simulink model "testmodel_1109"  (R2015b)
settings: Solver=FixedStepDiscrete  StartTime=0.0  StopTime=50  FixedStep=Ts  RelTol=1e-3
PreLoadFcn:
  | Ts_IO601 = 0.001;
InitFcn:
  | Ts_IO601 = 0.001;
  | Ts=0.004;
undefined symbols (not defined in the file or in its folder): DiscIntNeverNeededParam
libraries: canmsglib x13, speedgoatlib_IO601 x9, slrtlib x5, simulink x3
settings Model: Creator=lab2  LastModifiedBy=mohit
settings SolverCC: EnableConcurrentExecution=on
settings DataIOCC: SaveFormat=Array
settings OptimizationCC: BlockReduction=off  OptimizeBlockIOStorage=off  BufferReuse=off  GlobalBufferReuse=off  ExpressionFolding=off  LocalBlockOutputs=off
settings DebuggingCC: UnconnectedInputMsg=none  UnconnectedOutputMsg=none  UnconnectedLineMsg=none
settings HardwareCC: ProdBitPerPointer=32  ProdLargestAtomicFloat=None  ProdWordSize=32  ProdLongLongMode=on  ProdHWDeviceType=Generic->32-bit x86 compatible
settings RTWCC: SystemTargetFile=slrt.tlc  TemplateMakefile=slrt_default_tmf  Description=Simulink Real-Time  RTWCompilerOptimization=on
settings TargetCC: CodeReplacementLibrary=XPC_BLAS  ParMdlRefBuildCompliant=on  ConcurrentExecutionCompliant=on  GeneratePreprocessorConditionals=Use local settings  MatFileLogging=on  MATLABClassNameForMDSCustomization=xpcAperiodicCustomization
settings ConfigComp: CovModelRefEnable=Off

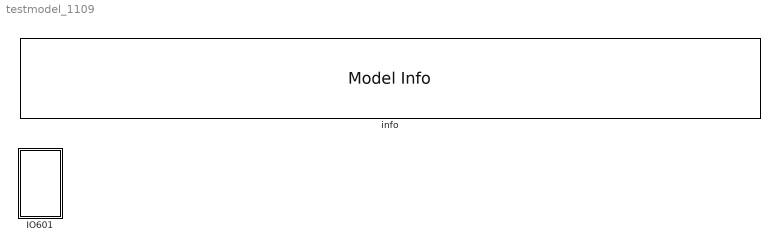
== system testmodel_1109 ==
  IO601 : Subsystem
  info : simulink/Model-Wide Utilities/Model Info  Frame=on  DisplayStringWithTags=|  HorizontalTextAlignment=Left  LeftAlignmentValue=0.02  SourceBlockDiagram=testmodel_1109  TagMaxNumber=20
      | SPEEDGOAT Simulink Real-Time  test model for Real-time target machine (SN2820)
      | prepared by Speedgoat with MATLAB R2015a
      | 
      | Build date: %<Created>

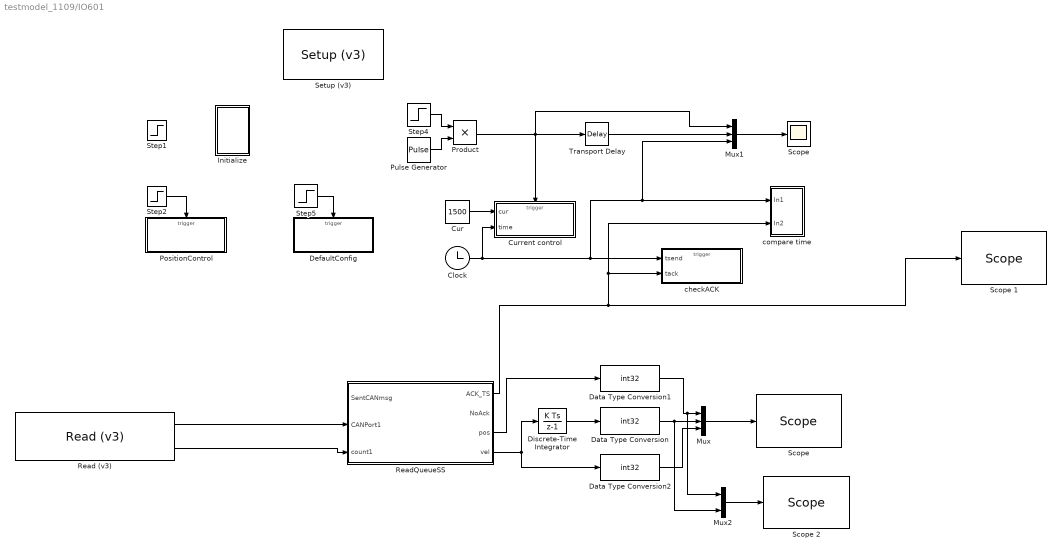
== system testmodel_1109/IO601 ==
  Clock : Clock
  Cur : Constant  Value=1500  OutMin=-1500  OutMax=1500  OutDataTypeStr=int32
  Current control : Subsystem  TreatAsAtomicUnit=on
  Data Type Conversion : DataTypeConversion  OutDataTypeStr=int32
  Data Type Conversion1 : DataTypeConversion  OutDataTypeStr=int32
  Data Type Conversion2 : DataTypeConversion  OutDataTypeStr=int32
  DefaultConfig : Subsystem  TreatAsAtomicUnit=on
  Discrete-Time Integrator : DiscreteIntegrator  InitialConditionSetting=State (most efficient)  SampleTime=-1  ICPrevOutput=DiscIntNeverNeededParam  ICPrevScaledInput=DiscIntNeverNeededParam
  Initialize : Subsystem
  Mux : Mux  Inputs=3
  Mux1 : Mux  Inputs=3
  Mux2 : Mux  Inputs=2
  "PositionControl " : Subsystem  TreatAsAtomicUnit=on
  Product : Product
  Pulse Generator : DiscretePulseGenerator  PulseType=Time based  Period=Ts*10  PulseWidth=10  PhaseDelay=10  SampleTime=Ts_IO601
  Read (v3) : speedgoatlib_IO601/Read (v3)  id=1  outputFormat=Vector of CAN_MESSAGE  port1=on  port2=off  depth1=37  depth2=4  sampletime=Ts  pciSlot=-1
  ReadQueueSS : Subsystem
  Scope : Scope
  "Scope " : slrtlib/Displays and Logging/Scope   scopeno=3  scopetype=Target  autostart=on  viewmode=Graphical sliding  formatstr='%15.6f'  grid=on  ylimits=[-90000,90000]  nosamples=50/Ts  noprepostsamples=0  interleave=1  triggermode=FreeRun  triggersignal=1  trigsignalfromport=off  triggerlevel=0.0  triggerslope=Either  triggerscope=1  triggersample=0  filename=data.dat  mode=Lazy  writesize=512  autorestart=off  dynamicfilemode=off  maxwritefilesize=512*1024^2
  Scope 1 : slrtlib/Displays and Logging/Scope   scopeno=12  scopetype=Target  autostart=on  viewmode=Graphical sliding  formatstr='%15.6f'  grid=on  ylimits=[0,125000]  nosamples=50/Ts  noprepostsamples=0  interleave=1  triggermode=FreeRun  triggersignal=1  trigsignalfromport=on  triggerlevel=0.0  triggerslope=Either  triggerscope=1  triggersample=0  filename=data.dat  mode=Lazy  writesize=512  autorestart=off  dynamicfilemode=off  maxwritefilesize=512*1024^2
  Scope 2 : slrtlib/Displays and Logging/Scope   scopeno=1  scopetype=File  autostart=on  viewmode=Graphical sliding  formatstr='%15.6f'  grid=on  ylimits=[-90000,90000]  nosamples=50/Ts  noprepostsamples=0  interleave=1  triggermode=FreeRun  triggersignal=1  trigsignalfromport=off  triggerlevel=0.0  triggerslope=Either  triggerscope=1  triggersample=0  filename=pos_vel.dat  mode=Lazy  writesize=512  autorestart=off  dynamicfilemode=off  maxwritefilesize=512*1024^2
  Setup (v3) : speedgoatlib_IO601/Setup (v3)  id=1  can1enable=on  can1bus=Highspeed  can1Baudrate=1 MBaud  can1UserBR=[1,1,5,2]  stdAcc1=[0,0,0,0]  extAcc1=[0,0,0,0]  can2enable=on  can2bus=Highspeed  can2Baudrate=1 MBaud  can2UserBR=[1,1,5,2]  stdAcc2=[0,0,0,0]  extAcc2=[0,0,0,0]  pciSlot=-1
  Step1 : Step  Time=10  SampleTime=Ts
  Step2 : Step  Time=25  SampleTime=Ts
  Step4 : Step  Time=14  Before=1  After=0  SampleTime=0
  Step5 : Step  Time=15  SampleTime=Ts
  Transport Delay : TransportDelay  DelayTime=Ts*10
  checkACK : Subsystem
  compare time : Subsystem
  wires:
  Step4/1 -> Product/1
  Pulse Generator/1 -> Product/2
  ReadQueueSS/1(ACK_TS) -> compare time/2(In2), checkACK/2(tack), Scope 1/1
  Cur/1 -> Current control/1(cur)
  Read (v3)/1 -> ReadQueueSS/2(CANPort1)
  Read (v3)/2 -> ReadQueueSS/3(count1)
  Step2/1 -> "PositionControl "/Trigger
  Product/1 -> Mux1/1, Transport Delay/1, Current control/Trigger
  Clock/1 -> Mux1/3, compare time/1(In1), checkACK/1(tsend), Current control/2(time)
  ReadQueueSS/4(vel) -> Discrete-Time Integrator/1, Data Type Conversion2/1
  Mux/1 -> "Scope "/1
  Discrete-Time Integrator/1 -> Data Type Conversion/1
  Data Type Conversion/1 -> Mux2/2, Mux/2
  Data Type Conversion1/1 -> Mux2/1, Mux/1
  Data Type Conversion2/1 -> Mux/3
  Transport Delay/1 -> Mux1/2
  Mux1/1 -> Scope/1
  Mux2/1 -> Scope 2/1
  ReadQueueSS/3(pos) -> Data Type Conversion1/1
  Step5/1 -> DefaultConfig/Trigger

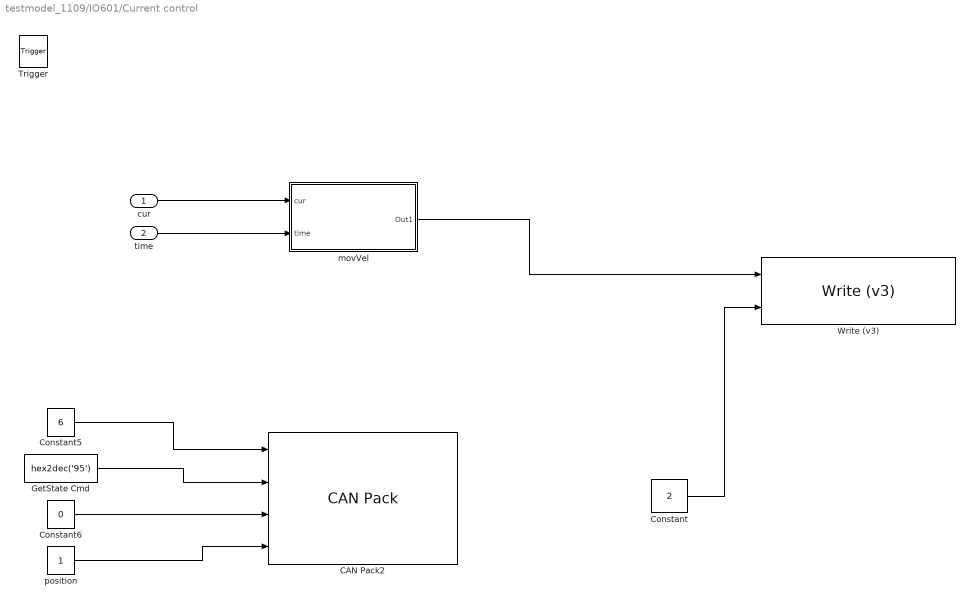
== system testmodel_1109/IO601/Current control ==
  cur : Inport
  time : Inport  Port=2
  Trigger : TriggerPort
  CAN Pack2 : canmsglib/CAN Pack  MsgList=(none)  MsgName=GetState  MsgIDType=Standard (11-bit identifier)  MsgIdentifier=hex2dec('503')  MsgLength=7  SignalInfo=Signal1$0$8$1$2$1$0$1$0$-Inf$Inf$#Signal2$8$8$1$2$1$0$1$0$-Inf$Inf$#time$16$32$1$2$1$0$1$0$-Inf$Inf$#mode$48$8$1$2$1$0$1$0$-Inf$Inf$#  NSignals=4  StartBits=str2num('[int32(0);int32(8);int32(16);int32(48)]')  SignalSizes=str2num('[int32(8);int32(8);int32(32);int32(8)]')  ByteOrders=str2num('[int32(1);int32(1);int32(1);int32(1)]')  DataTypes=str2num('[int32(2);int32(2);int32(2);int32(2)]')  MultiplexTypes=str2num('[int32(1);int32(1);int32(1);int32(1)]')  MultiplexValues=str2num('[double(0);double(0);double(0);double(0)]')  Factors=str2num('[double(1);double(1);double(1);double(1)]')  Offsets=str2num('[double(0);double(0);double(0);double(0)]')  Minimums=str2num('[double(-Inf);double(-Inf);double(-Inf);double(-Inf)]')  Maximums=str2num('[double(Inf);double(Inf);double(Inf);double(Inf)]')  Remote=off
      settings: DataFormat=manually specified signals
  Constant : Constant  Value=2
  Constant5 : Constant  Value=6
  Constant6 : Constant  Value=0
  GetState Cmd : Constant  Value=hex2dec('95')
  Write (v3) : speedgoatlib_IO601/Write (v3)  Priority=1  id=1  sampletime=-1  pciSlot=-1  inputType=CAN_MESSAGE plus count  port=1  maxMsg=2  status=on  init=[]  term=[]
  movVel : Subsystem
  position : Constant  OutDataTypeStr=uint8
  wires:
  Constant/1 -> Write (v3)/2
  Constant6/1 -> CAN Pack2/3
  Constant5/1 -> CAN Pack2/1
  GetState Cmd/1 -> CAN Pack2/2
  position/1 -> CAN Pack2/4
  cur/1 -> movVel/1(cur)
  time/1 -> movVel/2(time)
  movVel/1(Out1) -> Write (v3)/1

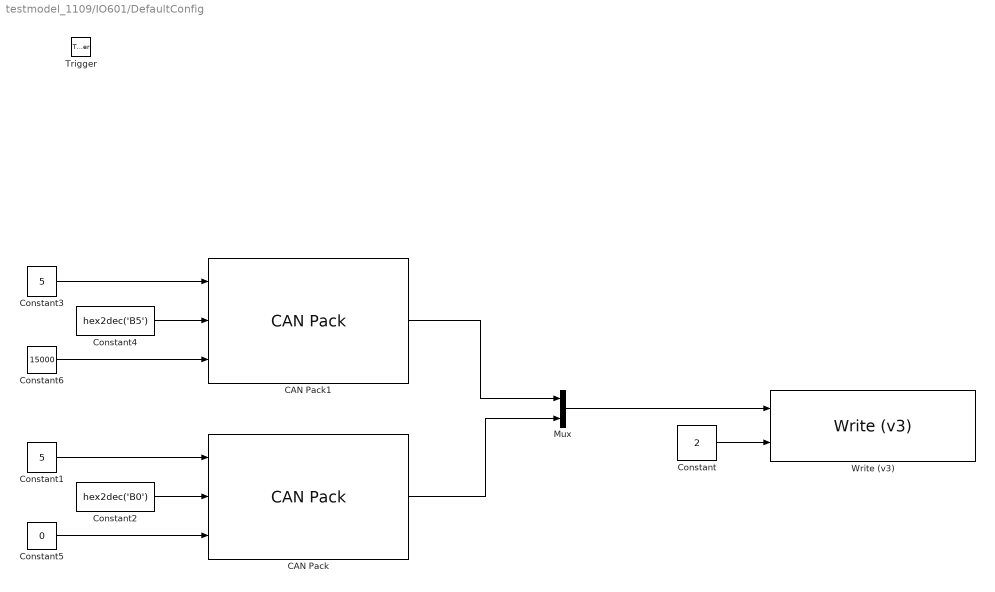
== system testmodel_1109/IO601/DefaultConfig ==
  Trigger : TriggerPort
  CAN Pack : canmsglib/CAN Pack  MsgList=(none)  MsgName=Position Msg  MsgIDType=Standard (11-bit identifier)  MsgIdentifier=hex2dec('503')  MsgLength=6  SignalInfo=Signal1$0$8$1$2$1$0$1$0$-Inf$Inf$#Signal2$8$8$1$2$1$0$1$0$-Inf$Inf$#Signal3$16$32$1$1$1$0$1$0$-Inf$Inf$#  NSignals=3  StartBits=str2num('[int32(0);int32(8);int32(16)]')  SignalSizes=str2num('[int32(8);int32(8);int32(32)]')  ByteOrders=str2num('[int32(1);int32(1);int32(1)]')  DataTypes=str2num('[int32(2);int32(2);int32(1)]')  MultiplexTypes=str2num('[int32(1);int32(1);int32(1)]')  MultiplexValues=str2num('[double(0);double(0);double(0)]')  Factors=str2num('[double(1);double(1);double(1)]')  Offsets=str2num('[double(0);double(0);double(0)]')  Minimums=str2num('[double(-Inf);double(-Inf);double(-Inf)]')  Maximums=str2num('[double(Inf);double(Inf);double(Inf)]')  Remote=off
      settings: DataFormat=manually specified signals
  CAN Pack1 : canmsglib/CAN Pack  MsgList=(none)  MsgName=Position Msg  MsgIDType=Standard (11-bit identifier)  MsgIdentifier=hex2dec('503')  MsgLength=6  SignalInfo=Signal1$0$8$1$2$1$0$1$0$-Inf$Inf$#Signal2$8$8$1$2$1$0$1$0$-Inf$Inf$#Signal3$16$32$1$1$1$0$1$0$-Inf$Inf$#  NSignals=3  StartBits=str2num('[int32(0);int32(8);int32(16)]')  SignalSizes=str2num('[int32(8);int32(8);int32(32)]')  ByteOrders=str2num('[int32(1);int32(1);int32(1)]')  DataTypes=str2num('[int32(2);int32(2);int32(1)]')  MultiplexTypes=str2num('[int32(1);int32(1);int32(1)]')  MultiplexValues=str2num('[double(0);double(0);double(0)]')  Factors=str2num('[double(1);double(1);double(1)]')  Offsets=str2num('[double(0);double(0);double(0)]')  Minimums=str2num('[double(-Inf);double(-Inf);double(-Inf)]')  Maximums=str2num('[double(Inf);double(Inf);double(Inf)]')  Remote=off
      settings: DataFormat=manually specified signals
  Constant : Constant  Value=2
  Constant1 : Constant  Value=5
  Constant2 : Constant  Value=hex2dec('B0')
  Constant3 : Constant  Value=5
  Constant4 : Constant  Value=hex2dec('B5')
  Constant5 : Constant  Value=0
  Constant6 : Constant  Value=15000
  Mux : Mux  Inputs=2
  Write (v3) : speedgoatlib_IO601/Write (v3)  Priority=1  id=1  sampletime=-1  pciSlot=-1  inputType=CAN_MESSAGE plus count  port=1  maxMsg=2  status=off  init=[]  term=[]
  wires:
  CAN Pack/1 -> Mux/2
  Constant/1 -> Write (v3)/2
  Constant1/1 -> CAN Pack/1
  Constant2/1 -> CAN Pack/2
  Constant5/1 -> CAN Pack/3
  CAN Pack1/1 -> Mux/1
  Constant3/1 -> CAN Pack1/1
  Constant4/1 -> CAN Pack1/2
  Constant6/1 -> CAN Pack1/3
  Mux/1 -> Write (v3)/1

== system testmodel_1109/IO601/Initialize ==
  GetState(ms) : Subsystem  TreatAsAtomicUnit=on
  InitialPosition : Subsystem  TreatAsAtomicUnit=on
  QuitError : Subsystem  TreatAsAtomicUnit=on
  Step : Step  SampleTime=Ts
  Step1 : Step  Time=2  SampleTime=Ts
  Step3 : Step  Time=2  SampleTime=Ts
  wires:
  Step/1 -> QuitError/Trigger
  Step3/1 -> InitialPosition/Trigger
  Step1/1 -> GetState(ms)/Trigger

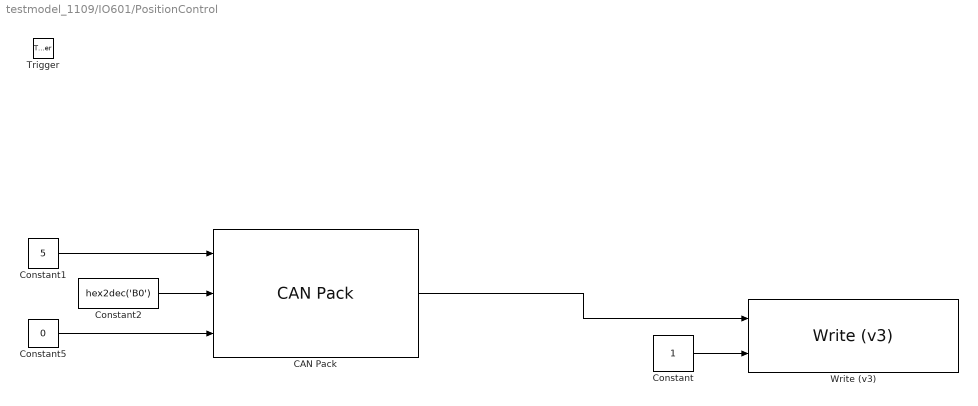
== system testmodel_1109/IO601/PositionControl  ==
  Trigger : TriggerPort
  CAN Pack : canmsglib/CAN Pack  MsgList=(none)  MsgName=Position Msg  MsgIDType=Standard (11-bit identifier)  MsgIdentifier=hex2dec('503')  MsgLength=6  SignalInfo=Signal1$0$8$1$2$1$0$1$0$-Inf$Inf$#Signal2$8$8$1$2$1$0$1$0$-Inf$Inf$#Signal3$16$32$1$1$1$0$1$0$-Inf$Inf$#  NSignals=3  StartBits=str2num('[int32(0);int32(8);int32(16)]')  SignalSizes=str2num('[int32(8);int32(8);int32(32)]')  ByteOrders=str2num('[int32(1);int32(1);int32(1)]')  DataTypes=str2num('[int32(2);int32(2);int32(1)]')  MultiplexTypes=str2num('[int32(1);int32(1);int32(1)]')  MultiplexValues=str2num('[double(0);double(0);double(0)]')  Factors=str2num('[double(1);double(1);double(1)]')  Offsets=str2num('[double(0);double(0);double(0)]')  Minimums=str2num('[double(-Inf);double(-Inf);double(-Inf)]')  Maximums=str2num('[double(Inf);double(Inf);double(Inf)]')  Remote=off
      settings: DataFormat=manually specified signals
  Constant : Constant
  Constant1 : Constant  Value=5
  Constant2 : Constant  Value=hex2dec('B0')
  Constant5 : Constant  Value=0
  Write (v3) : speedgoatlib_IO601/Write (v3)  Priority=1  id=1  sampletime=-1  pciSlot=-1  inputType=CAN_MESSAGE plus count  port=1  maxMsg=1  status=off  init=[]  term=[]
  wires:
  CAN Pack/1 -> Write (v3)/1
  Constant/1 -> Write (v3)/2
  Constant1/1 -> CAN Pack/1
  Constant2/1 -> CAN Pack/2
  Constant5/1 -> CAN Pack/3

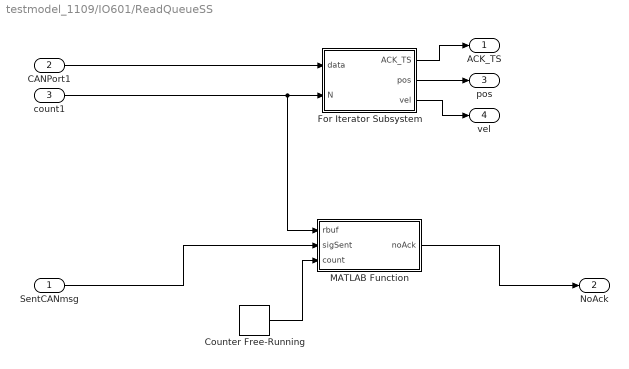
== system testmodel_1109/IO601/ReadQueueSS ==
  SentCANmsg : Inport
  CANPort1 : Inport  Port=2
  count1 : Inport  Port=3
  Counter Free-Running : simulink/Sources/Counter Free-Running  NumBits=2  tsamp=-1
  For Iterator Subsystem : Subsystem  TreatAsAtomicUnit=on
  MATLAB Function : MATLAB Function  TreatAsAtomicUnit=on
  ACK_TS : Outport
  " NoAck" : Outport  Port=2
  pos : Outport  Port=3
  vel : Outport  Port=4
  wires:
  CANPort1/1 -> For Iterator Subsystem/1(data)
  count1/1 -> MATLAB Function/1(rbuf), For Iterator Subsystem/2(N)
  For Iterator Subsystem/1(ACK_TS) -> ACK_TS/1
  Counter Free-Running/1 -> MATLAB Function/3(count)
  SentCANmsg/1 -> MATLAB Function/2(sigSent)
  MATLAB Function/1(noAck) -> " NoAck"/1
  For Iterator Subsystem/2(pos) -> pos/1
  For Iterator Subsystem/3(vel) -> vel/1

== system testmodel_1109/IO601/checkACK ==
  tsend : Inport
  tack : Inport  Port=2
  Trigger : TriggerPort
  MATLAB Function : MATLAB Function  TreatAsAtomicUnit=on
  STOP : Subsystem  TreatAsAtomicUnit=on
  wires:
  MATLAB Function/1(stop) -> STOP/1(stop)
  tack/1 -> MATLAB Function/2(tack)
  tsend/1 -> MATLAB Function/1(tsend)

== system testmodel_1109/IO601/compare time ==
  In1 : Inport
  In2 : Inport  Port=2
  Mux2 : Mux  Inputs=2
  Scope 2 : slrtlib/Displays and Logging/Scope   scopeno=50  scopetype=Target  autostart=on  viewmode=Graphical sliding  formatstr='%15.6f'  grid=on  ylimits=[0,125000]  nosamples=50/Ts  noprepostsamples=0  interleave=1  triggermode=FreeRun  triggersignal=1  trigsignalfromport=on  triggerlevel=0.0  triggerslope=Either  triggerscope=1  triggersample=0  filename=data.dat  mode=Lazy  writesize=512  autorestart=off  dynamicfilemode=off  maxwritefilesize=512*1024^2
  wires:
  Mux2/1 -> Scope 2/1
  In1/1 -> Mux2/1
  In2/1 -> Mux2/2

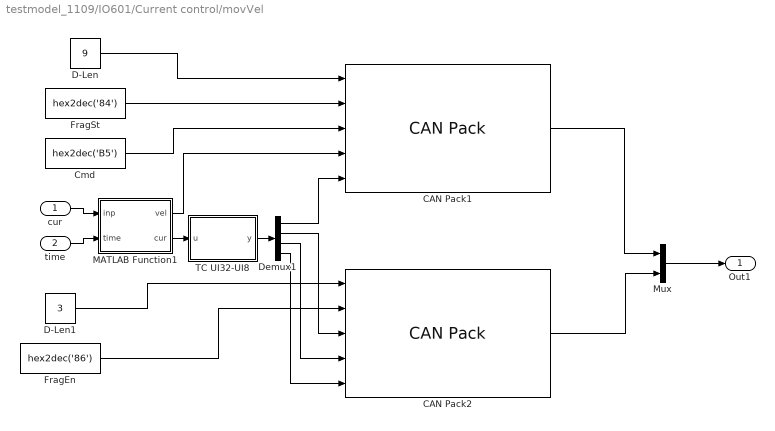
== system testmodel_1109/IO601/Current control/movVel ==
  cur : Inport
  time : Inport  Port=2
  CAN Pack1 : canmsglib/CAN Pack  MsgList=(none)  MsgName=Position Msg  MsgIDType=Standard (11-bit identifier)  MsgIdentifier=hex2dec('503')  MsgLength=8  SignalInfo=Signal1$0$8$1$2$1$0$1$0$-Inf$Inf$#Signal2$8$8$1$2$1$0$1$0$-Inf$Inf$#Signal3$16$8$1$2$1$0$1$0$-Inf$Inf$#Signal4$24$32$1$1$1$0$1$0$-Inf$Inf$#Signal5$56$8$1$2$1$0$1$0$-Inf$Inf$#  NSignals=5  StartBits=str2num('[int32(0);int32(8);int32(16);int32(24);int32(56)]')  SignalSizes=str2num('[int32(8);int32(8);int32(8);int32(32);int32(8)]')  ByteOrders=str2num('[int32(1);int32(1);int32(1);int32(1);int32(1)]')  DataTypes=str2num('[int32(2);int32(2);int32(2);int32(1);int32(2)]')  MultiplexTypes=str2num('[int32(1);int32(1);int32(1);int32(1);int32(1)]')  MultiplexValues=str2num('[double(0);double(0);double(0);double(0);double(0)]')  Factors=str2num('[double(1);double(1);double(1);double(1);double(1)]')  Offsets=str2num('[double(0);double(0);double(0);double(0);double(0)]')  Minimums=str2num('[double(-Inf);double(-Inf);double(-Inf);double(-Inf);double(-Inf)]')  Maximums=str2num('[double(Inf);double(Inf);double(Inf);double(Inf);double(Inf)]')  Remote=off
      settings: DataFormat=manually specified signals
  CAN Pack2 : canmsglib/CAN Pack  MsgList=(none)  MsgName=Position Msg  MsgIDType=Standard (11-bit identifier)  MsgIdentifier=hex2dec('503')  MsgLength=5  SignalInfo=Signal1$0$8$1$2$1$0$1$0$-Inf$Inf$#Signal2$8$8$1$2$1$0$1$0$-Inf$Inf$#Signal3$16$8$1$2$1$0$1$0$-Inf$Inf$#Signal4$24$8$1$2$1$0$1$0$-Inf$Inf$#Signal5$32$8$1$2$1$0$1$0$-Inf$Inf$#  NSignals=5  StartBits=str2num('[int32(0);int32(8);int32(16);int32(24);int32(32)]')  SignalSizes=str2num('[int32(8);int32(8);int32(8);int32(8);int32(8)]')  ByteOrders=str2num('[int32(1);int32(1);int32(1);int32(1);int32(1)]')  DataTypes=str2num('[int32(2);int32(2);int32(2);int32(2);int32(2)]')  MultiplexTypes=str2num('[int32(1);int32(1);int32(1);int32(1);int32(1)]')  MultiplexValues=str2num('[double(0);double(0);double(0);double(0);double(0)]')  Factors=str2num('[double(1);double(1);double(1);double(1);double(1)]')  Offsets=str2num('[double(0);double(0);double(0);double(0);double(0)]')  Minimums=str2num('[double(-Inf);double(-Inf);double(-Inf);double(-Inf);double(-Inf)]')  Maximums=str2num('[double(Inf);double(Inf);double(Inf);double(Inf);double(Inf)]')  Remote=off
      settings: DataFormat=manually specified signals
  Cmd : Constant  Value=hex2dec('B5')
  D-Len : Constant  Value=9
  D-Len1 : Constant  Value=3
  Demux1 : Demux
  FragEn : Constant  Value=hex2dec('86')
  FragSt : Constant  Value=hex2dec('84')
  MATLAB Function1 : MATLAB Function  TreatAsAtomicUnit=on
  Mux : Mux  Inputs=2
  TC UI32-UI8 : MATLAB Function  TreatAsAtomicUnit=on
  Out1 : Outport
  wires:
  D-Len/1 -> CAN Pack1/1
  Cmd/1 -> CAN Pack1/3
  CAN Pack1/1 -> Mux/1
  Mux/1 -> Out1/1
  FragSt/1 -> CAN Pack1/2
  FragEn/1 -> CAN Pack2/2
  D-Len1/1 -> CAN Pack2/1
  CAN Pack2/1 -> Mux/2
  MATLAB Function1/2(cur) -> TC UI32-UI8/1(u)
  Demux1/1 -> CAN Pack1/5
  Demux1/2 -> CAN Pack2/3
  Demux1/3 -> CAN Pack2/4
  Demux1/4 -> CAN Pack2/5
  cur/1 -> MATLAB Function1/1(inp)
  time/1 -> MATLAB Function1/2(time)
  MATLAB Function1/1(vel) -> CAN Pack1/4
  TC UI32-UI8/1(y) -> Demux1/1

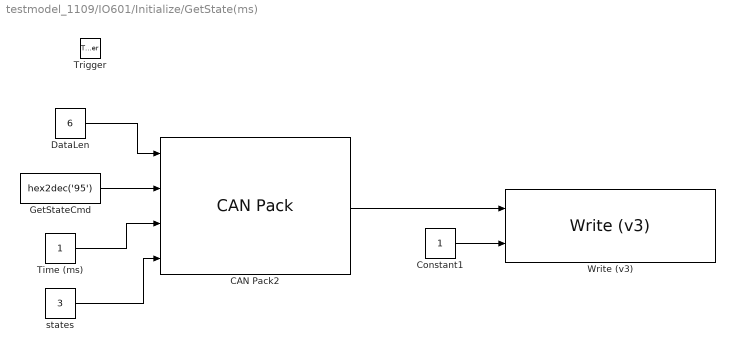
== system testmodel_1109/IO601/Initialize/GetState(ms) ==
  Trigger : TriggerPort
  CAN Pack2 : canmsglib/CAN Pack  MsgList=(none)  MsgName=GetState  MsgIDType=Standard (11-bit identifier)  MsgIdentifier=hex2dec('503')  MsgLength=7  SignalInfo=Signal1$0$8$1$2$1$0$1$0$-Inf$Inf$#Signal2$8$8$1$2$1$0$1$0$-Inf$Inf$#time$16$32$1$2$1$0$1$0$-Inf$Inf$#mode$48$8$1$2$1$0$1$0$-Inf$Inf$#  NSignals=4  StartBits=str2num('[int32(0);int32(8);int32(16);int32(48)]')  SignalSizes=str2num('[int32(8);int32(8);int32(32);int32(8)]')  ByteOrders=str2num('[int32(1);int32(1);int32(1);int32(1)]')  DataTypes=str2num('[int32(2);int32(2);int32(2);int32(2)]')  MultiplexTypes=str2num('[int32(1);int32(1);int32(1);int32(1)]')  MultiplexValues=str2num('[double(0);double(0);double(0);double(0)]')  Factors=str2num('[double(1);double(1);double(1);double(1)]')  Offsets=str2num('[double(0);double(0);double(0);double(0)]')  Minimums=str2num('[double(-Inf);double(-Inf);double(-Inf);double(-Inf)]')  Maximums=str2num('[double(Inf);double(Inf);double(Inf);double(Inf)]')  Remote=off
      settings: DataFormat=manually specified signals
  Constant1 : Constant
  DataLen : Constant  Value=6
  GetStateCmd : Constant  Value=hex2dec('95')
  Time (ms) : Constant
  Write (v3) : speedgoatlib_IO601/Write (v3)  Priority=1  id=1  sampletime=-1  pciSlot=-1  inputType=CAN_MESSAGE plus count  port=1  maxMsg=1  status=off  init=[]  term=[]
  states : Constant  Value=3  OutDataTypeStr=uint8
  wires:
  Constant1/1 -> Write (v3)/2
  Time (ms)/1 -> CAN Pack2/3
  DataLen/1 -> CAN Pack2/1
  GetStateCmd/1 -> CAN Pack2/2
  CAN Pack2/1 -> Write (v3)/1
  states/1 -> CAN Pack2/4

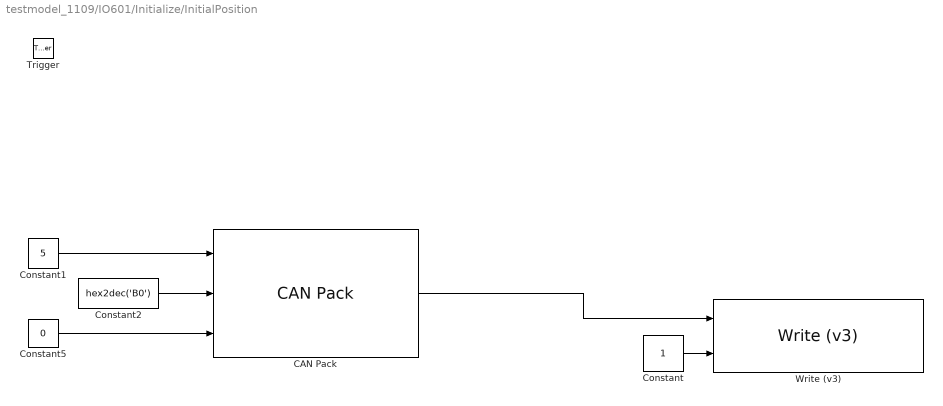
== system testmodel_1109/IO601/Initialize/InitialPosition ==
  Trigger : TriggerPort
  CAN Pack : canmsglib/CAN Pack  MsgList=(none)  MsgName=Position Msg  MsgIDType=Standard (11-bit identifier)  MsgIdentifier=1283  MsgLength=6  SignalInfo=Signal1$0$8$1$2$1$0$1$0$-Inf$Inf$#Signal2$8$8$1$2$1$0$1$0$-Inf$Inf$#Signal3$16$32$1$1$1$0$1$0$-Inf$Inf$#  NSignals=3  StartBits=str2num('[int32(0);int32(8);int32(16)]')  SignalSizes=str2num('[int32(8);int32(8);int32(32)]')  ByteOrders=str2num('[int32(1);int32(1);int32(1)]')  DataTypes=str2num('[int32(2);int32(2);int32(1)]')  MultiplexTypes=str2num('[int32(1);int32(1);int32(1)]')  MultiplexValues=str2num('[double(0);double(0);double(0)]')  Factors=str2num('[double(1);double(1);double(1)]')  Offsets=str2num('[double(0);double(0);double(0)]')  Minimums=str2num('[double(-Inf);double(-Inf);double(-Inf)]')  Maximums=str2num('[double(Inf);double(Inf);double(Inf)]')  Remote=off
      settings: DataFormat=manually specified signals
  Constant : Constant
  Constant1 : Constant  Value=5
  Constant2 : Constant  Value=hex2dec('B0')
  Constant5 : Constant  Value=0
  Write (v3) : speedgoatlib_IO601/Write (v3)  Priority=1  id=1  sampletime=-1  pciSlot=-1  inputType=CAN_MESSAGE plus count  port=1  maxMsg=1  status=off  init=[]  term=[]
  wires:
  CAN Pack/1 -> Write (v3)/1
  Constant/1 -> Write (v3)/2
  Constant1/1 -> CAN Pack/1
  Constant2/1 -> CAN Pack/2
  Constant5/1 -> CAN Pack/3

== system testmodel_1109/IO601/Initialize/QuitError ==
  Trigger : TriggerPort
  CAN Pack : canmsglib/CAN Pack  MsgList=(none)  MsgName=QuitError  MsgIDType=Standard (11-bit identifier)  MsgIdentifier=hex2dec('503')  MsgLength=2  SignalInfo=Signal1$0$8$1$2$1$0$1$0$-Inf$Inf$#Signal2$8$8$1$2$1$0$1$0$-Inf$Inf$#  NSignals=2  StartBits=str2num('[int32(0);int32(8)]')  SignalSizes=str2num('[int32(8);int32(8)]')  ByteOrders=str2num('[int32(1);int32(1)]')  DataTypes=str2num('[int32(2);int32(2)]')  MultiplexTypes=str2num('[int32(1);int32(1)]')  MultiplexValues=str2num('[double(0);double(0)]')  Factors=str2num('[double(1);double(1)]')  Offsets=str2num('[double(0);double(0)]')  Minimums=str2num('[double(-Inf);double(-Inf)]')  Maximums=str2num('[double(Inf);double(Inf)]')  Remote=off
      settings: DataFormat=manually specified signals
  Constant1 : Constant
  Constant2 : Constant
  Constant3 : Constant  Value=139
  Write (v3) : speedgoatlib_IO601/Write (v3)  Priority=1  id=1  sampletime=-1  pciSlot=-1  inputType=CAN_MESSAGE plus count  port=1  maxMsg=1  status=off  init=[]  term=[]
  wires:
  Constant3/1 -> CAN Pack/2
  Constant2/1 -> CAN Pack/1
  CAN Pack/1 -> Write (v3)/1
  Constant1/1 -> Write (v3)/2

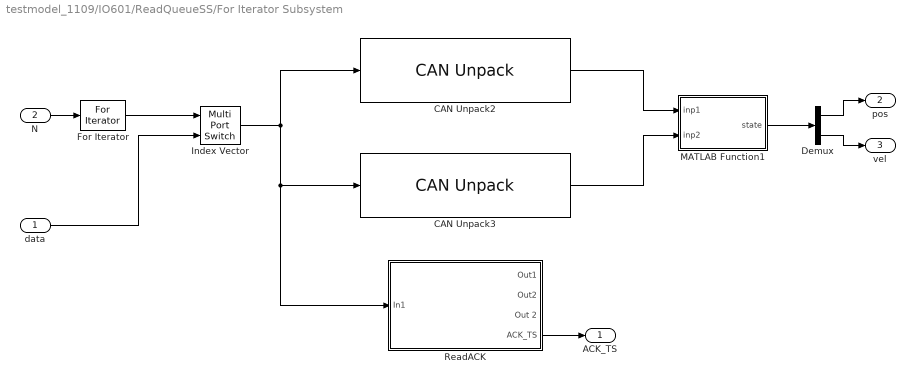
== system testmodel_1109/IO601/ReadQueueSS/For Iterator Subsystem ==
  data : Inport
  N : Inport  Port=2
  CAN Unpack2 : canmsglib/CAN Unpack  MsgList=(none)  MsgName=CANGSraw  MsgIDType=Standard (11-bit identifier)  MsgIdentifier=hex2dec('703')  MsgLength=8  SignalInfo=DLen$0$8$1$2$1$0$1$0$-Inf$Inf$#Cmd$8$8$1$2$1$0$1$0$-Inf$Inf$#Position$16$32$1$1$1$0$1$0$-Inf$Inf$#  NSignals=3  IDPort=off  TimestampPort=off  ErrorPort=off  RemotePort=off  LengthPort=off  StatusPort=off  StartBits=str2num('[int32(0);int32(8);int32(16)]')  SignalSizes=str2num('[int32(8);int32(8);int32(32)]')  ByteOrders=str2num('[int32(1);int32(1);int32(1)]')  DataTypes=str2num('[int32(2);int32(2);int32(1)]')  MultiplexTypes=str2num('[int32(1);int32(1);int32(1)]')  MultiplexValues=str2num('[double(0);double(0);double(0)]')  Factors=str2num('[double(1);double(1);double(1)]')  Offsets=str2num('[double(0);double(0);double(0)]')  Minimums=str2num('[double(-Inf);double(-Inf);double(-Inf)]')  Maximums=str2num('[double(Inf);double(Inf);double(Inf)]')
      settings: DataFormat=raw data
  CAN Unpack3 : canmsglib/CAN Unpack  MsgList=(none)  MsgName=CANGSraw2  MsgIDType=Standard (11-bit identifier)  MsgIdentifier=hex2dec('703')  MsgLength=7  SignalInfo=DLen$0$8$1$2$1$0$1$0$-Inf$Inf$#Cmd$8$8$1$2$1$0$1$0$-Inf$Inf$#Position$16$32$1$1$1$0$1$0$-Inf$Inf$#  NSignals=3  IDPort=off  TimestampPort=off  ErrorPort=off  RemotePort=off  LengthPort=off  StatusPort=off  StartBits=str2num('[int32(0);int32(8);int32(16)]')  SignalSizes=str2num('[int32(8);int32(8);int32(32)]')  ByteOrders=str2num('[int32(1);int32(1);int32(1)]')  DataTypes=str2num('[int32(2);int32(2);int32(1)]')  MultiplexTypes=str2num('[int32(1);int32(1);int32(1)]')  MultiplexValues=str2num('[double(0);double(0);double(0)]')  Factors=str2num('[double(1);double(1);double(1)]')  Offsets=str2num('[double(0);double(0);double(0)]')  Minimums=str2num('[double(-Inf);double(-Inf);double(-Inf)]')  Maximums=str2num('[double(Inf);double(Inf);double(Inf)]')
      settings: DataFormat=raw data
  Demux : Demux  Outputs=2
  For Iterator : ForIterator  IterationSource=external  IterationLimit=20  IterationVariableDataType=int8
  Index Vector : MultiPortSwitch  Inputs=1
  MATLAB Function1 : MATLAB Function  TreatAsAtomicUnit=on
  ReadACK : Subsystem
  ACK_TS : Outport
  pos : Outport  Port=2
  vel : Outport  Port=3
  wires:
  For Iterator/1 -> Index Vector/1
  data/1 -> Index Vector/2
  N/1 -> For Iterator/1
  Index Vector/1 -> ReadACK/1(In1), CAN Unpack3/1, CAN Unpack2/1
  CAN Unpack2/1 -> MATLAB Function1/1(inp1)
  CAN Unpack3/1 -> MATLAB Function1/2(inp2)
  MATLAB Function1/1(state) -> Demux/1
  Demux/1 -> pos/1
  Demux/2 -> vel/1
  ReadACK/4(ACK_TS) -> ACK_TS/1

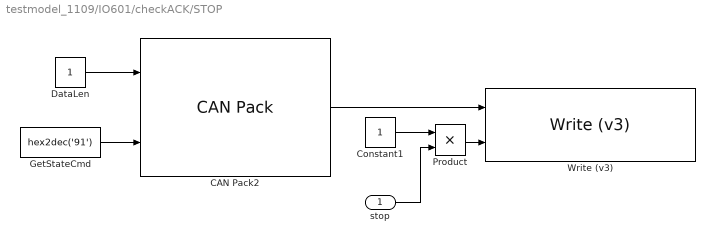
== system testmodel_1109/IO601/checkACK/STOP ==
  stop : Inport
  CAN Pack2 : canmsglib/CAN Pack  MsgList=(none)  MsgName=GetState  MsgIDType=Standard (11-bit identifier)  MsgIdentifier=hex2dec('503')  MsgLength=2  SignalInfo=Signal1$0$8$1$2$1$0$1$0$-Inf$Inf$#Signal2$8$8$1$2$1$0$1$0$-Inf$Inf$#  NSignals=2  StartBits=str2num('[int32(0);int32(8)]')  SignalSizes=str2num('[int32(8);int32(8)]')  ByteOrders=str2num('[int32(1);int32(1)]')  DataTypes=str2num('[int32(2);int32(2)]')  MultiplexTypes=str2num('[int32(1);int32(1)]')  MultiplexValues=str2num('[double(0);double(0)]')  Factors=str2num('[double(1);double(1)]')  Offsets=str2num('[double(0);double(0)]')  Minimums=str2num('[double(-Inf);double(-Inf)]')  Maximums=str2num('[double(Inf);double(Inf)]')  Remote=off
      settings: DataFormat=manually specified signals
  Constant1 : Constant
  DataLen : Constant
  GetStateCmd : Constant  Value=hex2dec('91')
  Product : Product
  Write (v3) : speedgoatlib_IO601/Write (v3)  Priority=1  id=1  sampletime=-1  pciSlot=-1  inputType=CAN_MESSAGE plus count  port=1  maxMsg=1  status=off  init=[]  term=[]
  wires:
  DataLen/1 -> CAN Pack2/1
  GetStateCmd/1 -> CAN Pack2/2
  CAN Pack2/1 -> Write (v3)/1
  Constant1/1 -> Product/1
  Product/1 -> Write (v3)/2
  stop/1 -> Product/2

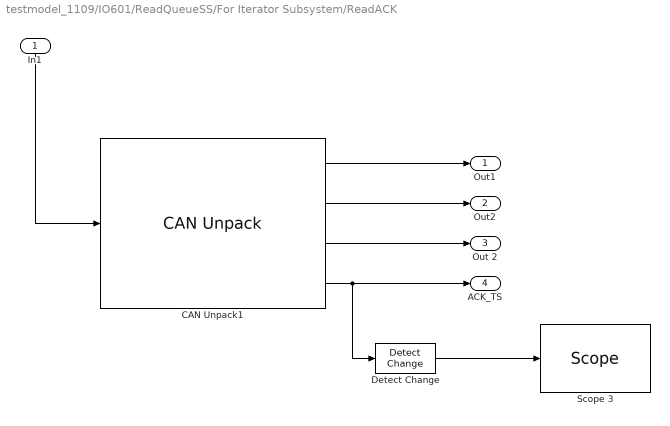
== system testmodel_1109/IO601/ReadQueueSS/For Iterator Subsystem/ReadACK ==
  In1 : Inport
  CAN Unpack1 : canmsglib/CAN Unpack  MsgList=(none)  MsgName=Message21  MsgIDType=Standard (11-bit identifier)  MsgIdentifier=hex2dec('703')  MsgLength=4  SignalInfo=DLen$0$8$1$2$1$0$1$0$-Inf$Inf$#Cmd$8$8$1$2$1$0$1$0$-Inf$Inf$#Param$16$16$1$1$1$0$1$0$-Inf$Inf$#  NSignals=3  IDPort=off  TimestampPort=on  ErrorPort=off  RemotePort=off  LengthPort=off  StatusPort=off  StartBits=str2num('[int32(0);int32(8);int32(16)]')  SignalSizes=str2num('[int32(8);int32(8);int32(16)]')  ByteOrders=str2num('[int32(1);int32(1);int32(1)]')  DataTypes=str2num('[int32(2);int32(2);int32(1)]')  MultiplexTypes=str2num('[int32(1);int32(1);int32(1)]')  MultiplexValues=str2num('[double(0);double(0);double(0)]')  Factors=str2num('[double(1);double(1);double(1)]')  Offsets=str2num('[double(0);double(0);double(0)]')  Minimums=str2num('[double(-Inf);double(-Inf);double(-Inf)]')  Maximums=str2num('[double(Inf);double(Inf);double(Inf)]')
  Detect Change : simulink/Logic and Bit Operations/Detect Change  vinit=0  InputProcessing=Inherited  OutDataTypeStr=boolean
  Scope 3 : slrtlib/Displays and Logging/Scope   scopeno=10  scopetype=Target  autostart=on  viewmode=Graphical sliding  formatstr='%15.6f'  grid=on  ylimits=[0000,0000]  nosamples=50/Ts  noprepostsamples=0  interleave=1  triggermode=FreeRun  triggersignal=1  trigsignalfromport=off  triggerlevel=0.0  triggerslope=Either  triggerscope=1  triggersample=0  filename=data.dat  mode=Lazy  writesize=512  autorestart=off  dynamicfilemode=off  maxwritefilesize=512*1024^2
  Out1 : Outport
  Out2 : Outport  Port=2
  Out 2 : Outport  Port=3
  ACK_TS : Outport  Port=4
  wires:
  CAN Unpack1/3 -> Out 2/1
  CAN Unpack1/2 -> Out2/1
  CAN Unpack1/4 -> Detect Change/1, ACK_TS/1
  Detect Change/1 -> Scope 3/1
  CAN Unpack1/1 -> Out1/1
  In1/1 -> CAN Unpack1/1

== matlab function testmodel_1109/IO601/ReadQueueSS/MATLAB Function ==
  data: rbuf input; sigSent input; noAck output; count input
function noAck = checkACK(rbuf, sigSent, count)
%#codegen
noAck = 0;
if sigSent
    if rbuf == 0 && count == 4
        noAck = 1;
    else
        noAck = 0;
    end
end
end

== matlab function testmodel_1109/IO601/ReadQueueSS/For Iterator Subsystem/MATLAB Function1 ==
  data: inp1 input; state output int32 size=[1 2]; inp2 input
function state    = decrypt_gs_pv(inp1, inp2)
%#codegen

persistent stitched;
persistent pos;
persistent vel;

if isempty(stitched)
   stitched = zeros(1,12);
   pos = zeros(1,4);
   vel = zeros(1,4);
end

if inp1(3) == hex2dec('95')
    stitched(1) = inp1(1);
    pos(1:4) = uint8(inp1(4:7));
    if inp1(1) > 8
        vel(1) = uint8(inp1(8));
        vel(2:4) = uint8(inp2(3:5));
    end
end
pos1 = typecast(uint8(pos), 'int32');
vel1 = typecast(uint8(vel), 'int32');

state = [pos1 vel1];
end

== matlab function testmodel_1109/IO601/Current control/movVel/MATLAB Function1 ==
  data: vel output int32; cur output uint32 size=1; inp input int32; time input
function [vel, cur] = fcn(inp, time)
%#codegen

c = inp*sin(2*pi*100/time);
% c = inp

if c > 0
    vel = int32(90000);
else
    vel = int32(-90000);
end
c1 = (abs(c));
cur = uint32(c1);
end

== matlab function testmodel_1109/IO601/checkACK/MATLAB Function ==
  data: tsend input; stop output; tack input
function stop = fcn(tsend, tack)
%#codegen
stop = 0;
tdiff = abs(tsend-tack);
persistent count;
if isempty(count)
    count = 0;
end

if tdiff > 0.04
    count = count+1;
else
    count = 0;
end

if count >= 5
   stop = 1;
else
    stop = 0;
end
end

== matlab function testmodel_1109/IO601/Current control/movVel/TC UI32-UI8 ==
  data: u input uint32; y output uint8 size=[1 4]
function y = tc_ui32toui8(u)
%#codegen
y = typecast(uint32(u), 'uint8');
